simulink model "PID_Loop_2024a"  (R2024b)
settings: Solver=FixedStepAuto  StartTime=0.0  StopTime=tspan  FixedStep=dt  RelTol=1e-3
model workspace (MAT data in the model file):
  Drag_Constants = 1
  mass = [5.51 5.51 5.51 1 1 1]
  mass_6a = [5 5 5 1 1 1]
values from neighbouring files (symbols this model uses):
  acc_bias_instability = 19e-6*9.81    (= 0.00018639)    [init.m]
  acc_noise = 60e-6*9.81    (= 0.0005886)    [init.m]
  acc_vel_rw = 0.02/sqrt(3600)    [init.m]
  do_bouyancy_flag = 1    [PID_testing_data_producer.m]    (also in init.m = 0)
  do_gravity_flag = 1    [PID_testing_data_producer.m]    (also in init.m = 0)
  do_imu_noise_flag = 0    [PID_testing_data_producer.m]    (also in init.m)
  dt = 0.001    [PID_testing_data_producer.m]    (also in init.m)
  Dt = 0.01    [init.m]
  g = 9.8067    [constants.m]    (also in constants.mat = 9.80665)
  gyro_bias_instability = 1.5/3600/360    (= 1.15740740741e-06)    [init.m]
  gyro_noise = 5e-3*2*pi/360    (= 8.72664625997e-05)    [init.m]
  gyro_rw = 0.16*2*pi/360/sqrt(3600)    [init.m]
  H = [1 0 0 ... (first row only)    [init.m]
  inverse_wrench = pinv(wrench)    [calculate_wrench.m]    (also in constants.m = geometry_properties.inverse_wrench; geometry_properties.mat = [0.09 0.09 -0.09 -0.09 0.353553390593 0.353553390593 0.35355)
  mag_noise = 0.1    [init.m]
  max_pitch_torque = norm(wrench*(F_max*[1 1 -1 -1 0 0 0 0]'))    [calculate_wrench.m]
  max_roll_torque = norm(wrench*(F_max*[1 -1 1 -1 0 0 0 0]'))    [calculate_wrench.m]
  max_yaw_torque = norm(wrench*(F_max*[0 0 0 0 -1 1 -1 1]'))    [calculate_wrench.m]
  pitch_force = [0         0         0         0    1.0000         0]    [constants.m]
  plot_dt = 0.01    [init.m]
  Q = diag([0.0001, 0.0001, 0.1])    [init.m]
  R = [.1 0 ... (first row only)    [init.m]
  roll_force = [0         0         0    0.5000         0         0]    [constants.m]
  states_desired = [x_des;E_des]    [init.m]
  volume = 0.0074    [constants.m]    (also in constants.mat = 0.0073741788)
  volume_center = [0, 0, 0.1]    [constants.m]    (also in constants.mat = [0 0 0.1])
  water_density = 997    [constants.m]    (also in constants.mat = 1000)
  waypoints = input_state_errors(:,i)    [PID_testing_data_producer.m]    (also in init.m = [0, 0, 0])
  wrench = eval(w)    [calculate_wrench.m]    (also in constants.m = geometry_properties.wrench; constants.mat = [0 0 0 0 -0.7071 -0.7071 -0.7071 -0.7071 0 0 0 0 ... (48 ele; geometry_properties.mat = [0 0 -1 0.22 0.25 0 0 0 -1 -0.22 0.25 0 ... (48 elements, 6x; wrench.m)
  x_force = [0.4100         0         0         0         0         0]    [constants.m]    (also in init2.m = [0.410000000000000	0	0	0	0	0])
  y_force = [0    0.5000         0         0         0         0]    [constants.m]    (also in init2.m = [0	0.500000000000000	0	0	0	0])
  yaw_force = [0         0         0         0         0    0.5000]    [constants.m]
  z_force = [0         0    1.2500         0         0         0]    [constants.m]
undefined symbols (not defined in the file or in its folder): E0_est, fractalcoef, IMU, P, v0_e_est, x0_e_est
libraries: slpidlib x4, mspsensorlib x2, shared6dof x1, simulink x1, sharedTrackingLibrary x1, uavutilslib x1
(part 1 of 2)
settings Model: Creator=zenyn  LastModifiedBy=vinso
settings DataIOCC: LoggingToFile=on
settings OptimizationCC: EnhancedBackFolding=on  PassReuseOutputArgsAs=Individual arguments  ZeroExternalMemoryAtStartup=off  ZeroInternalMemoryAtStartup=off  MaxStackSize=64  OptimizeBlockOrder=speed  DifferentSizesBufferReuse=on  OptimizationCustomize=off  EfficientTunableParamExpr=on
settings DebuggingCC: ParameterTunabilityLossMsg=error
settings SFSimCC: MATLABDynamicMemAlloc=off
settings RTWCC: Description=Embedded Coder  SystemTargetFile=ert.tlc  HardwareBoard=Robot Operating System 2 (ROS 2)  TLCOptions="-aInlineSetEventsForThisBaseRateFcn=TLC_FALSE -aSuppressMultiTaskScheduler=TLC_FALSE  -aRateBasedStepFcn=0"  TemplateMakefile=ert_default_tmf  Toolchain=Colcon Tools  TargetLang=C++
settings CodeAppCC: ForceParamTrailComments=on  IgnoreCustomStorageClasses=off  OperatorAnnotations=on  SimulinkDataObjDesc=on  SFDataObjDesc=on  InsertBlockDesc=on
settings ERTTargetCC: CodeInterfacePackaging=C++ class  InlinedParameterPlacement=Hierarchical  RootIOFormat=Structure reference  DynamicArrayContainerType=coder::array

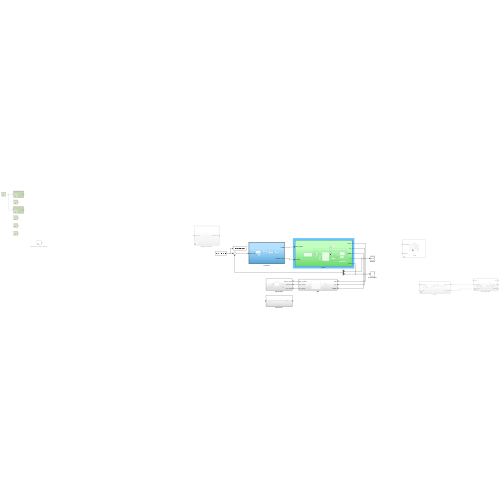
[thumbnail: Simulink's stored preview of the top-level diagram]
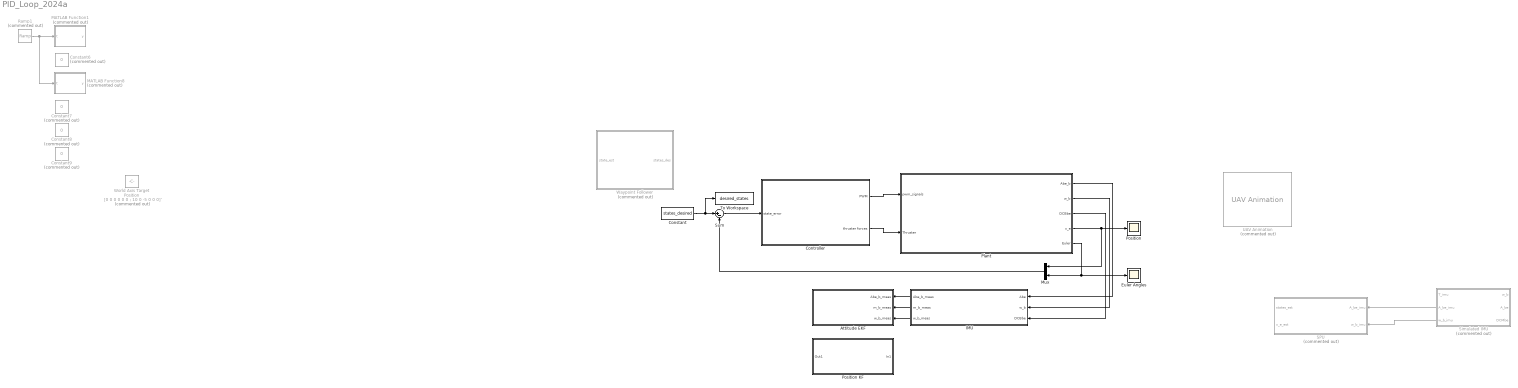
== system PID_Loop_2024a ==
  Attitude EKF : Subsystem
  Constant : Constant  Value=states_desired
  Constant{6..9} (4 alike) : Constant  Commented=on  Value=0
  Controller : Subsystem  TreatAsAtomicUnit=on
  Euler Angles : Scope
  IMU : Subsystem
  MATLAB Function1 : MATLAB Function  Commented=on  TreatAsAtomicUnit=on
  MATLAB Function8 : MATLAB Function  Commented=on  TreatAsAtomicUnit=on
  Mux : Mux  Inputs=2
  Plant : Subsystem
  Position : Scope
  Position KF : Subsystem
  Ramp1 : simulink/Sources/Ramp  Commented=on  slope=1  start=0  InitialOutput=0
  SPU : Subsystem  Commented=on
  Simulated IMU : Subsystem  Commented=on
  Sum : Sum  Inputs=|+-
  To Workspace : ToWorkspace  VariableName=desired_states  SaveFormat=Timeseries  SampleTime=Dt
  UAV Animation : uavutilslib/UAV Animation  Commented=on  NumUAV=1  DynamicUAVConfig=off  UAVType=FixedWing  UAVSize=1  UAVColor=[1 0 0]  UAVTrajectoryAlpha=1  InertialZDirection=Down  RotationFormat=Quaternion  DrawMarkers=off  SampleTime=Dt
  Waypoint Follower : Subsystem  Commented=on
  World Axis Target Position : Constant  Commented=on  Value=[0 0 0 0 0 0 ; 10 0 -5 0 0 0]'
  wires:
  Ramp1/1 -> MATLAB Function8/1(t), MATLAB Function1/1(t)
  Simulated IMU/2(A_be_imu) -> SPU/1(A_be_imu)
  Simulated IMU/3(w_b_imu) -> SPU/2(w_b_imu)
  Constant/1 -> Sum/1, To Workspace/1
  Plant/4(x_e) -> Position/1, Mux/1
  Sum/1 -> Controller/1(state_error)
  IMU/1(Abe_b_meas) -> Attitude EKF/1(Abe_b_meas)
  IMU/2(m_b_meas) -> Attitude EKF/2(m_b_meas)
  IMU/3(w_b_meas) -> Attitude EKF/3(w_b_meas)
  Plant/1(Abe_b) -> IMU/1(Abe)
  Plant/3(DCBbe) -> IMU/3(DCBbe)
  Plant/2(w_b) -> IMU/2(w_b)
  Controller/2(thruster forces) -> Plant/2(Thruster)
  Controller/1(PWM) -> Plant/1(pwm_signals)
  Plant/5(Euler) -> Mux/2, Euler Angles/1
  Mux/1 -> Sum/2

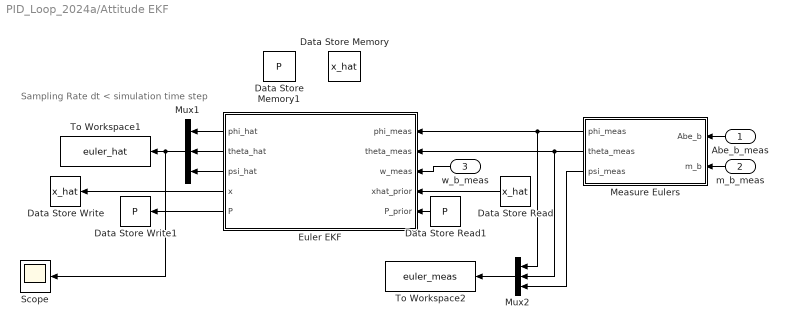
== system PID_Loop_2024a/Attitude EKF ==
  note: Sampling Rate dt < simulation time step
  Abe_b_meas : Inport
  m_b_meas : Inport  Port=2
  w_b_meas : Inport  Port=3
  Data Store Memory : DataStoreMemory  DataStoreName=x_hat  WriteAfterWriteMsg=warning  InitialValue=xhat0  ShowAdditionalParam=off
  Data Store Memory1 : DataStoreMemory  DataStoreName=P  WriteAfterWriteMsg=warning  InitialValue=P0  ShowAdditionalParam=off
  Data Store Read : DataStoreRead  DataStoreName=x_hat  IndexOptions=Index vector (dialog)  Indices=1  OutputSizes=1
  Data Store Read1 : DataStoreRead  DataStoreName=P  IndexOptions=Index vector (dialog)  Indices=1  OutputSizes=1
  Data Store Write : DataStoreWrite  DataStoreName=x_hat  IndexOptions=Index vector (dialog)  Indices=1  OutputSizes=1
  Data Store Write1 : DataStoreWrite  DataStoreName=P  IndexOptions=Index vector (dialog)  Indices=1  OutputSizes=1
  Euler EKF : MATLAB Function  TreatAsAtomicUnit=on
  Measure Eulers : MATLAB Function  TreatAsAtomicUnit=on
  Mux1 : Mux  Inputs=3
  Mux2 : Mux  Inputs=3
  Scope : Scope
  To Workspace1 : ToWorkspace  VariableName=euler_hat  SaveFormat=Timeseries  SampleTime=plot_dt
  To Workspace2 : ToWorkspace  VariableName=euler_meas  SaveFormat=Timeseries  SampleTime=plot_dt
  wires:
  Measure Eulers/1(phi_meas) -> Euler EKF/1(phi_meas), Mux2/1
  Euler EKF/4(x) -> Data Store Write/1
  Measure Eulers/2(theta_meas) -> Mux2/2, Euler EKF/2(theta_meas)
  Mux1/1 -> Scope/1, To Workspace1/1
  Data Store Read1/1 -> Euler EKF/5(P_prior)
  Euler EKF/1(phi_hat) -> Mux1/1
  Euler EKF/5(P) -> Data Store Write1/1
  Euler EKF/3(psi_hat) -> Mux1/3
  Euler EKF/2(theta_hat) -> Mux1/2
  Data Store Read/1 -> Euler EKF/4(xhat_prior)
  Abe_b_meas/1 -> Measure Eulers/1(Abe_b)
  Measure Eulers/3(psi_meas) -> Mux2/3
  Mux2/1 -> To Workspace2/1
  m_b_meas/1 -> Measure Eulers/2(m_b)
  w_b_meas/1 -> Euler EKF/3(w_meas)

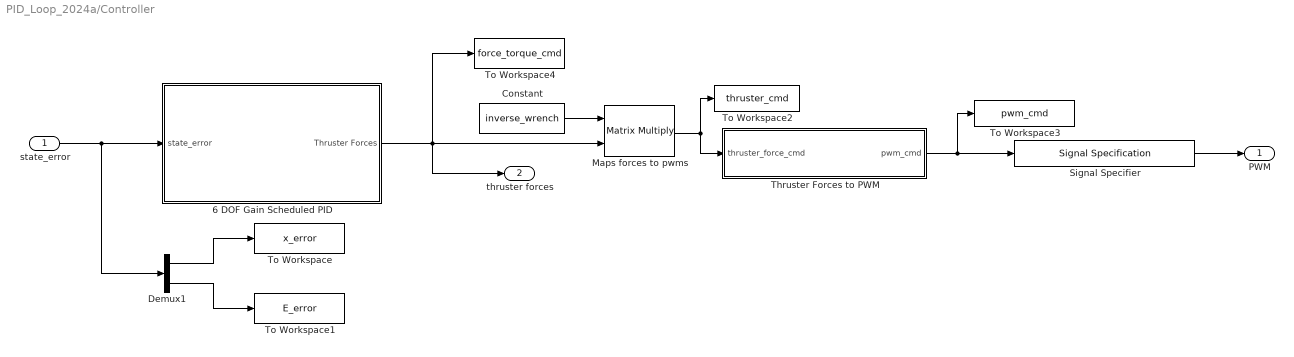
== system PID_Loop_2024a/Controller ==
  state_error : Inport
  6 DOF Gain Scheduled PID : Subsystem
  Constant : Constant  Value=inverse_wrench
  Demux1 : Demux  Outputs=2
  Maps forces to pwms : Product  Multiplication=Matrix(*)
  Signal Specifier : SignalSpecification  OutMin=[1200 ]  OutMax=[ 1800 ]  OutDataTypeStr=double  Unit=µs  Dimensions=[8 1]
  Thruster Forces to PWM : MATLAB Function  TreatAsAtomicUnit=on
  To Workspace : ToWorkspace  VariableName=x_error  SaveFormat=Timeseries  SampleTime=plot_dt
  To Workspace1 : ToWorkspace  VariableName=E_error  SaveFormat=Timeseries  SampleTime=plot_dt
  To Workspace2 : ToWorkspace  VariableName=thruster_cmd  SaveFormat=Timeseries  SampleTime=-1
  To Workspace3 : ToWorkspace  VariableName=pwm_cmd  SaveFormat=Timeseries  SampleTime=-1
  To Workspace4 : ToWorkspace  VariableName=force_torque_cmd  SaveFormat=Timeseries  SampleTime=plot_dt
  PWM : Outport
  thruster forces : Outport  Port=2
  wires:
  Thruster Forces to PWM/1(pwm_cmd) -> Signal Specifier/1, To Workspace3/1
  Signal Specifier/1 -> PWM/1
  Demux1/1 -> To Workspace/1
  Demux1/2 -> To Workspace1/1
  Maps forces to pwms/1 -> Thruster Forces to PWM/1(thruster_force_cmd), To Workspace2/1
  Constant/1 -> Maps forces to pwms/1
  state_error/1 -> 6 DOF Gain Scheduled PID/1(state_error), Demux1/1
  6 DOF Gain Scheduled PID/1(Thruster Forces) -> Maps forces to pwms/2, thruster forces/1, To Workspace4/1

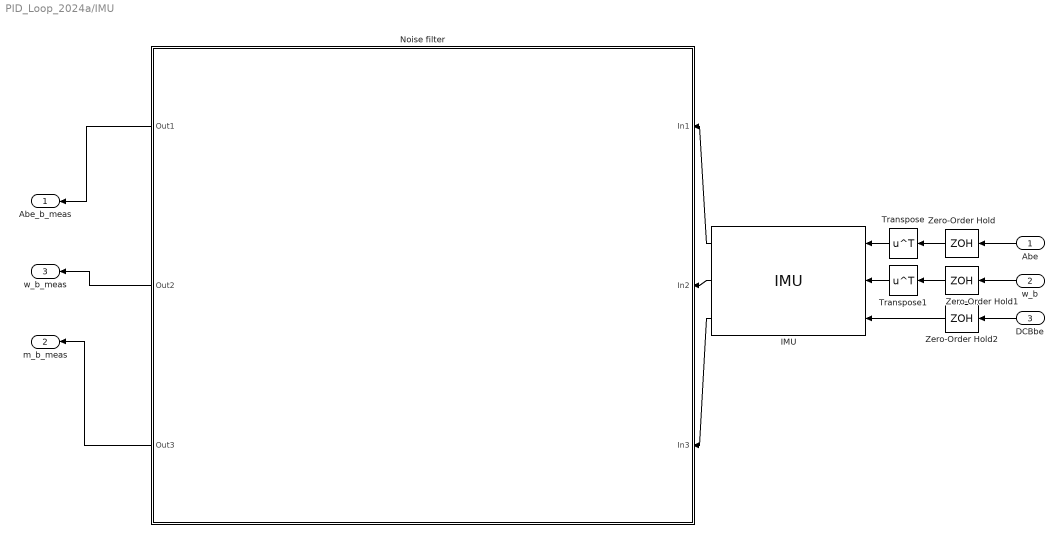
== system PID_Loop_2024a/IMU ==
  Abe : Inport
  w_b : Inport  Port=2
  DCBbe : Inport  Port=3
  IMU : mspsensorlib/IMU  DispRefFrame=NED  TemperaturePort=off  Temperature=25  MagneticFieldPort=off  MagneticFieldNED=[ 27.5550, -2.4169, -16.0849 ]  MagneticFieldENU=[ -2.4169, 27.5550, 16.0849 ]  SeedDouble=67  SimulateUsing=Interpreted execution  AccelParamsMeasurementRange=Inf  AccelParamsResolution=0  AccelParamsConstantBias=[ 0, 0, 0 ]  AccelParamsAxesMisalignment=[ 100, 0, 0; 0, 100, 0; 0, 0, 100 ]  AccelParamsNoiseDensity=acc_vel_rw*[ 1, 1, 1 ]  AccelParamsBiasInstability=acc_bias_instability*[ 1, 1, 1 ]  AccelParamsBiasInstabilityNumerator=fractalcoef().Numerator  AccelParamsBiasInstabilityDenominator=fractalcoef().Denominator  AccelParamsRandomWalk=acc_noise*[1, 1, 1]  AccelParamsNoiseType=double-sided  AccelParamsTemperatureBias=[ 0, 0, 0 ]  AccelParamsTemperatureScaleFactor=[ 0, 0, 0 ]  GyroParamsMeasurementRange=Inf  GyroParamsResolution=0  GyroParamsConstantBias=[ 0, 0, 0 ]  GyroParamsAxesMisalignment=[ 100, 0, 0; 0, 100, 0; 0, 0, 100 ]  GyroParamsAccelerationBias=[ 0, 0, 0 ]  GyroParamsNoiseDensity=gyro_rw*[ 1, 1, 1 ]  GyroParamsBiasInstability=gyro_bias_instability*[ 1, 1, 1 ]  GyroParamsBiasInstabilityNumerator=fractalcoef().Numerator  GyroParamsBiasInstabilityDenominator=fractalcoef().Denominator  GyroParamsRandomWalk=gyro_noise*[1, 1, 1]  GyroParamsNoiseType=double-sided  GyroParamsTemperatureBias=[ 0, 0, 0 ]  GyroParamsTemperatureScaleFactor=[ 0, 0, 0 ]  MagParamsMeasurementRange=Inf  MagParamsResolution=0  MagParamsConstantBias=[ 0, 0, 0 ]  MagParamsAxesMisalignment=[ 100, 0, 0; 0, 100, 0; 0, 0, 100 ]  MagParamsNoiseDensity=mag_noise*[1, 1, 1]  MagParamsBiasInstability=[ 0, 0, 0 ]  MagParamsBiasInstabilityNumerator=fractalcoef().Numerator  MagParamsBiasInstabilityDenominator=fractalcoef().Denominator  MagParamsRandomWalk=[ 0, 0, 0 ]  MagParamsNoiseType=double-sided  MagParamsTemperatureBias=[ 0, 0, 0 ]  MagParamsTemperatureScaleFactor=[ 0, 0, 0 ]
  Noise filter : Subsystem
  Transpose : Math  Operator=transpose
  Transpose1 : Math  Operator=transpose
  Zero-Order Hold : ZeroOrderHold  SampleTime=dt
  Zero-Order Hold1 : ZeroOrderHold  SampleTime=dt
  Zero-Order Hold2 : ZeroOrderHold  SampleTime=dt
  Abe_b_meas : Outport
  m_b_meas : Outport  Port=2
  w_b_meas : Outport  Port=3
  wires:
  Transpose/1 -> IMU/1
  Zero-Order Hold2/1 -> IMU/3
  Zero-Order Hold/1 -> Transpose/1
  Transpose1/1 -> IMU/2
  Zero-Order Hold1/1 -> Transpose1/1
  w_b/1 -> Zero-Order Hold1/1
  Abe/1 -> Zero-Order Hold/1
  DCBbe/1 -> Zero-Order Hold2/1
  IMU/1 -> Noise filter/1(In1)
  IMU/2 -> Noise filter/2(In2)
  IMU/3 -> Noise filter/3(In3)
  Noise filter/1(Out1) -> Abe_b_meas/1
  Noise filter/2(Out2) -> w_b_meas/1
  Noise filter/3(Out3) -> m_b_meas/1

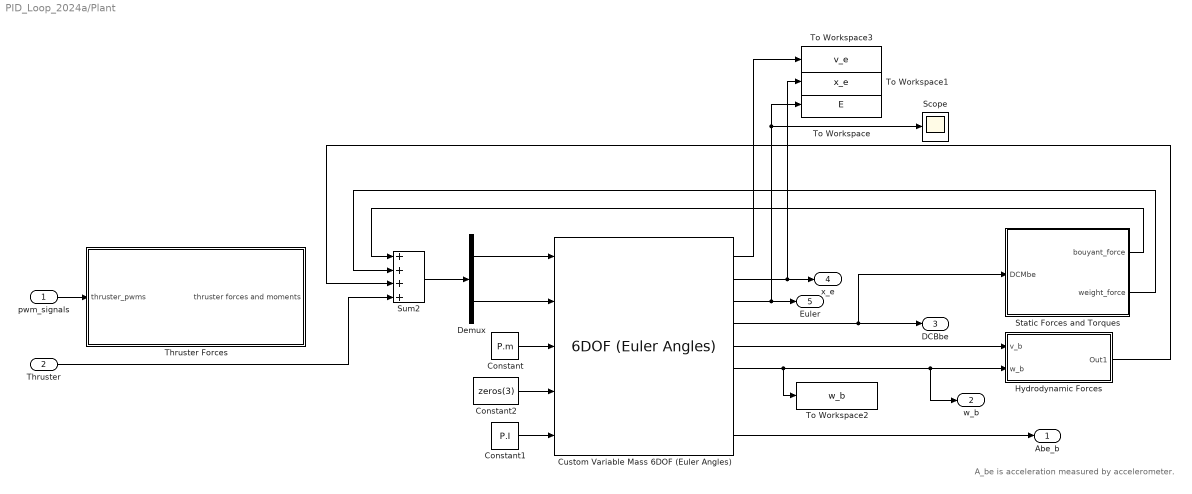
== system PID_Loop_2024a/Plant ==
  note: A_be is acceleration measured by accelerometer.
  pwm_signals : Inport  SampleTime=dt
  Thruster : Inport  Port=2
  Constant : Constant  Value=P.m
  Constant1 : Constant  Value=P.I
  Constant2 : Constant  Value=zeros(3)
  Custom Variable Mass 6DOF (Euler Angles) : shared6dof/6DOF (Euler Angles)  units=Metric (MKS)  mtype=Custom Variable  rep=Euler Angles  xme_0=x0_e  Vm_0=v0_e  eul_0=E0  pm_0=w0  mass_0=1.0  mass_e=0.5  mass_f=2.0  inertia=eye(3)  inertia_e=eye(3)  inertia_f=2*eye(3)  k_quat=1.0  vre_flag=off  abi_flag=on  aMode=0  xme_statename=''  Vm_statename=''  eul_statename=''  quat_statename=''  pm_statename=''  mass_statename=''
      settings: LibrarySourceBlock=aerolib6dof2/Custom Variable Mass 6DOF (Euler Angles)
  Demux : Demux  Outputs=2
  Hydrodynamic Forces : Subsystem
  Scope : Scope
  Static Forces and Torques : Subsystem
  Sum2 : Sum  Inputs=++++
  Thruster Forces : Subsystem
  To Workspace : ToWorkspace  VariableName=E  SaveFormat=Timeseries  SampleTime=plot_dt
  To Workspace1 : ToWorkspace  VariableName=x_e  SaveFormat=Timeseries  SampleTime=plot_dt
  To Workspace2 : ToWorkspace  VariableName=w_b  SaveFormat=Timeseries  SampleTime=plot_dt
  To Workspace3 : ToWorkspace  VariableName=v_e  SaveFormat=Timeseries  SampleTime=plot_dt
  Abe_b : Outport  SampleTime=Dt
  w_b : Outport  Port=2  SampleTime=Dt
  DCBbe : Outport  Port=3  SampleTime=Dt
  x_e : Outport  Port=4
  Euler : Outport  Port=5
  wires:
  Custom Variable Mass 6DOF (Euler Angles)/9 -> Abe_b/1
  Constant/1 -> Custom Variable Mass 6DOF (Euler Angles)/3
  Constant1/1 -> Custom Variable Mass 6DOF (Euler Angles)/5
  Constant2/1 -> Custom Variable Mass 6DOF (Euler Angles)/4
  Custom Variable Mass 6DOF (Euler Angles)/5 -> Hydrodynamic Forces/1(v_b)
  Custom Variable Mass 6DOF (Euler Angles)/4 -> Static Forces and Torques/1(DCMbe), DCBbe/1
  pwm_signals/1 -> Thruster Forces/1(thruster_pwms)
  Hydrodynamic Forces/1(Out1) -> Sum2/3
  Static Forces and Torques/2(weight_force) -> Sum2/2
  Static Forces and Torques/1(bouyant_force) -> Sum2/1
  Custom Variable Mass 6DOF (Euler Angles)/6 -> To Workspace2/1, w_b/1, Hydrodynamic Forces/2(w_b)
  Demux/2 -> Custom Variable Mass 6DOF (Euler Angles)/2
  Demux/1 -> Custom Variable Mass 6DOF (Euler Angles)/1
  Custom Variable Mass 6DOF (Euler Angles)/3 -> Euler/1, Scope/1, To Workspace/1
  Custom Variable Mass 6DOF (Euler Angles)/2 -> To Workspace1/1, x_e/1
  Custom Variable Mass 6DOF (Euler Angles)/1 -> To Workspace3/1
  Sum2/1 -> Demux/1
  Thruster/1 -> Sum2/4

== system PID_Loop_2024a/Position KF ==
  In1 : Inport
  Out1 : Outport
  wires:
  In1/1 -> Out1/1

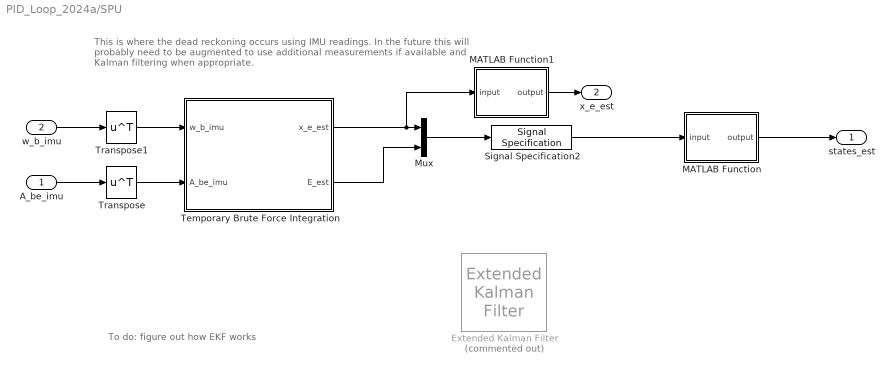
== system PID_Loop_2024a/SPU ==
  note: To do: figure out how EKF works
  note: This is where the dead reckoning occurs using IMU readings. In the future this will
      | probably need to be augmented to use additional measurements if available and
      | Kalman filtering when appropriate.
  A_be_imu : Inport
  w_b_imu : Inport  Port=2
  Extended Kalman Filter : sharedTrackingLibrary/Extended Kalman Filter  Commented=on  StateTransitionFcn=myStateTransitionFcn  HasStateTransitionJacobianFcn=off  HasAdditiveProcessNoise=Additive  ProcessNoise=1  HasTimeVaryingProcessNoise=off  HasStateTransitionFcnExtraArgument=0  InitialState=0  InitialStateCovariance=1  MeasurementFcn1=myMeasurementFcn  HasMeasurementJacobianFcn1=off  HasMeasurementEnablePort1=off  HasAdditiveMeasurementNoise1=Additive  MeasurementNoise1=1  HasTimeVaryingMeasurementNoise1=off  HasMeasurementFcnExtraArgument1=0  HasMeasurementWrapping1=off  MeasurementFcn2=myMeasurementFcn  HasMeasurementJacobianFcn2=off  HasMeasurementEnablePort2=off  HasAdditiveMeasurementNoise2=Additive  MeasurementNoise2=1  HasTimeVaryingMeasurementNoise2=off  HasMeasurementFcnExtraArgument2=0  HasMeasurementWrapping2=off  MeasurementFcn3=myMeasurementFcn  HasMeasurementJacobianFcn3=off  HasMeasurementEnablePort3=off  HasAdditiveMeasurementNoise3=Additive  MeasurementNoise3=1  HasTimeVaryingMeasurementNoise3=off  HasMeasurementFcnExtraArgument3=0  HasMeasurementWrapping3=off  MeasurementFcn4=myMeasurementFcn  HasMeasurementJacobianFcn4=off  HasMeasurementEnablePort4=off  HasAdditiveMeasurementNoise4=Additive  MeasurementNoise4=1  HasTimeVaryingMeasurementNoise4=off  HasMeasurementFcnExtraArgument4=0  HasMeasurementWrapping4=off  MeasurementFcn5=myMeasurementFcn  HasMeasurementJacobianFcn5=off  HasMeasurementEnablePort5=off  HasAdditiveMeasurementNoise5=Additive  MeasurementNoise5=1  HasTimeVaryingMeasurementNoise5=off  HasMeasurementFcnExtraArgument5=0  HasMeasurementWrapping5=off  EnableMultirate=off  StateTransitionFcnSampleTime=1  MeasurementFcn1SampleTime=1  MeasurementFcn2SampleTime=1  MeasurementFcn3SampleTime=1  MeasurementFcn4SampleTime=1  MeasurementFcn5SampleTime=1  UseCurrentEstimator=on  OutputStateCovariance=off  DataType=double  SampleTime=1  NumberOfMeasurements=1
  MATLAB Function : MATLAB Function  TreatAsAtomicUnit=on
  MATLAB Function1 : MATLAB Function  TreatAsAtomicUnit=on
  Mux : Mux  Inputs=2
  Signal Specification2 : SignalSpecification  Dimensions=[6 1]
  Temporary Brute Force Integration : Subsystem
  Transpose : Math  Operator=transpose
  Transpose1 : Math  Operator=transpose
  states_est : Outport
  x_e_est : Outport  Port=2
  wires:
  w_b_imu/1 -> Transpose1/1
  A_be_imu/1 -> Transpose/1
  Temporary Brute Force Integration/2(E_est) -> Mux/2
  Temporary Brute Force Integration/1(x_e_est) -> MATLAB Function1/1(input), Mux/1
  Mux/1 -> Signal Specification2/1
  Signal Specification2/1 -> MATLAB Function/1(input)
  Transpose1/1 -> Temporary Brute Force Integration/1(w_b_imu)
  Transpose/1 -> Temporary Brute Force Integration/2(A_be_imu)
  MATLAB Function/1(output) -> states_est/1
  MATLAB Function1/1(output) -> x_e_est/1

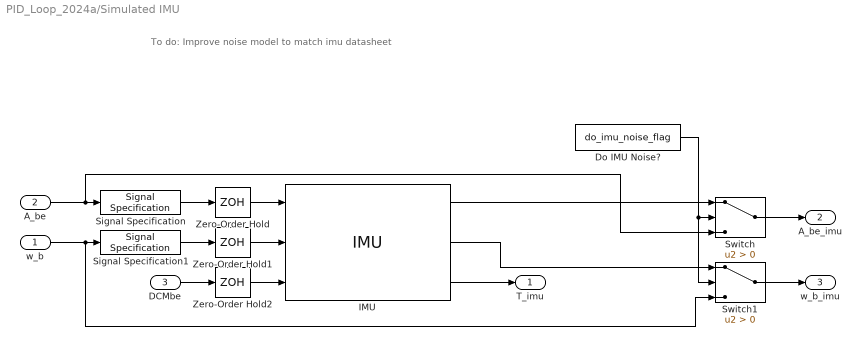
== system PID_Loop_2024a/Simulated IMU ==
  note: To do: Improve noise model to match imu datasheet
  w_b : Inport  SampleTime=Dt
  A_be : Inport  Port=2  SampleTime=Dt
  DCMbe : Inport  Port=3
  Do IMU Noise? : Constant  Value=do_imu_noise_flag
  IMU : mspsensorlib/IMU  DispRefFrame=NED  TemperaturePort=off  Temperature=25  MagneticFieldPort=off  MagneticFieldNED=[ 27.5550, -2.4169, -16.0849 ]  MagneticFieldENU=[ -2.4169, 27.5550, 16.0849 ]  SeedDouble=67  SimulateUsing=Interpreted execution  AccelParamsMeasurementRange=IMU.accelMaxRating  AccelParamsResolution=IMU.accelResolution  AccelParamsConstantBias=[ 0, 0, 0 ]  AccelParamsAxesMisalignment=[ 100, 0, 0; 0, 100, 0; 0, 0, 100 ]  AccelParamsNoiseDensity=[ IMU.accelVelRNDWalk, 0, 0 ]  AccelParamsBiasInstability=[ 0, 0, 0 ]  AccelParamsBiasInstabilityNumerator=fractalcoef().Numerator  AccelParamsBiasInstabilityDenominator=fractalcoef().Denominator  AccelParamsRandomWalk=[ 0, 0, 0 ]  AccelParamsNoiseType=double-sided  AccelParamsTemperatureBias=[ 0, 0, 0 ]  AccelParamsTemperatureScaleFactor=[ 0, 0, 0 ]  GyroParamsMeasurementRange=Inf  GyroParamsResolution=IMU.gyroResolution  GyroParamsConstantBias=[ 0, 0, 0 ]  GyroParamsAxesMisalignment=[ 100, 0, 0; 0, 100, 0; 0, 0, 100 ]  GyroParamsAccelerationBias=[ 0, 0, 0 ]  GyroParamsNoiseDensity=[ IMU.gyroAngleRNDWalk, 0, 0 ]  GyroParamsBiasInstability=[ 0, 0, 0 ]  GyroParamsBiasInstabilityNumerator=fractalcoef().Numerator  GyroParamsBiasInstabilityDenominator=fractalcoef().Denominator  GyroParamsRandomWalk=[ 0, 0, 0 ]  GyroParamsNoiseType=double-sided  GyroParamsTemperatureBias=[ 0, 0, 0 ]  GyroParamsTemperatureScaleFactor=[ 0, 0, 0 ]  MagParamsMeasurementRange=Inf  MagParamsResolution=IMU.magsResolution  MagParamsConstantBias=[ 0, 0, 0 ]  MagParamsAxesMisalignment=[ 100, 0, 0; 0, 100, 0; 0, 0, 100 ]  MagParamsNoiseDensity=[ 0, 0, 0 ]  MagParamsBiasInstability=[ 0, 0, 0 ]  MagParamsBiasInstabilityNumerator=fractalcoef().Numerator  MagParamsBiasInstabilityDenominator=fractalcoef().Denominator  MagParamsRandomWalk=[ 0, 0, 0 ]  MagParamsNoiseType=double-sided  MagParamsTemperatureBias=[ 0, 0, 0 ]  MagParamsTemperatureScaleFactor=[ 0, 0, 0 ]
  Signal Specification : SignalSpecification  Dimensions=[1 3]
  Signal Specification1 : SignalSpecification  Dimensions=[1 3]
  Switch : Switch  Criteria=u2 > Threshold  SaturateOnIntegerOverflow=off  InputSameDT=off
  Switch1 : Switch  Criteria=u2 > Threshold  SaturateOnIntegerOverflow=off  InputSameDT=off
  Zero-Order Hold : ZeroOrderHold  SampleTime=Dt
  Zero-Order Hold1 : ZeroOrderHold  SampleTime=Dt
  Zero-Order Hold2 : ZeroOrderHold  SampleTime=Dt
  T_imu : Outport
  A_be_imu : Outport  Port=2
  w_b_imu : Outport  Port=3
  wires:
  w_b/1 -> Switch1/3, Signal Specification1/1
  A_be/1 -> Switch/3, Signal Specification/1
  Signal Specification/1 -> Zero-Order Hold/1
  Signal Specification1/1 -> Zero-Order Hold1/1
  IMU/1 -> Switch/1
  IMU/2 -> Switch1/1
  IMU/3 -> T_imu/1
  DCMbe/1 -> Zero-Order Hold2/1
  Zero-Order Hold/1 -> IMU/1
  Zero-Order Hold1/1 -> IMU/2
  Zero-Order Hold2/1 -> IMU/3
  Do IMU Noise?/1 -> Switch1/2, Switch/2
  Switch/1 -> A_be_imu/1
  Switch1/1 -> w_b_imu/1

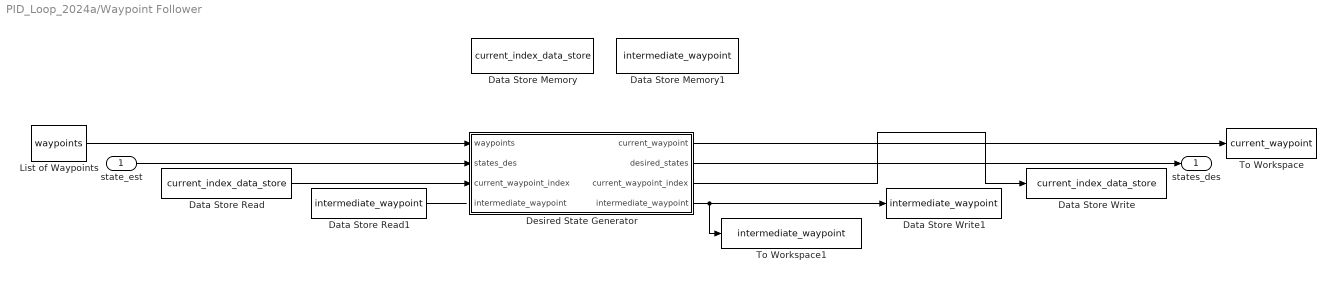
== system PID_Loop_2024a/Waypoint Follower ==
  state_est : Inport  SampleTime=Dt
  Data Store Memory : DataStoreMemory  DataStoreName=current_index_data_store  WriteAfterWriteMsg=warning  InitialValue=1  ShowAdditionalParam=off
  Data Store Memory1 : DataStoreMemory  DataStoreName=intermediate_waypoint  WriteAfterWriteMsg=warning  InitialValue=[9999,9999,9999]  ShowAdditionalParam=off
  Data Store Read : DataStoreRead  DataStoreName=current_index_data_store  IndexOptions=Index vector (dialog)  Indices=1  OutputSizes=1
  Data Store Read1 : DataStoreRead  DataStoreName=intermediate_waypoint  IndexOptions=Index vector (dialog)  Indices=1  OutputSizes=1
  Data Store Write : DataStoreWrite  DataStoreName=current_index_data_store  IndexOptions=Index vector (dialog)  Indices=1  OutputSizes=1
  Data Store Write1 : DataStoreWrite  DataStoreName=intermediate_waypoint  IndexOptions=Index vector (dialog)  Indices=1  OutputSizes=1
  Desired State Generator : MATLAB Function  TreatAsAtomicUnit=on
  List of Waypoints : Constant  Value=waypoints
  To Workspace : ToWorkspace  VariableName=current_waypoint  SaveFormat=Timeseries  SampleTime=-1
  To Workspace1 : ToWorkspace  VariableName=intermediate_waypoint  SaveFormat=Timeseries  SampleTime=-1
  states_des : Outport  SampleTime=Dt
  wires:
  state_est/1 -> Desired State Generator/2(states_des)
  Desired State Generator/2(desired_states) -> states_des/1
  Desired State Generator/3(current_waypoint_index) -> Data Store Write/1
  List of Waypoints/1 -> Desired State Generator/1(waypoints)
  Desired State Generator/1(current_waypoint) -> To Workspace/1
  Data Store Read/1 -> Desired State Generator/3("current_waypoint_index ")
  Data Store Read1/1 -> ?
  Desired State Generator/4(intermediate_waypoint) -> Data Store Write1/1, To Workspace1/1
  ? -> Desired State Generator/4("intermediate_waypoint ")

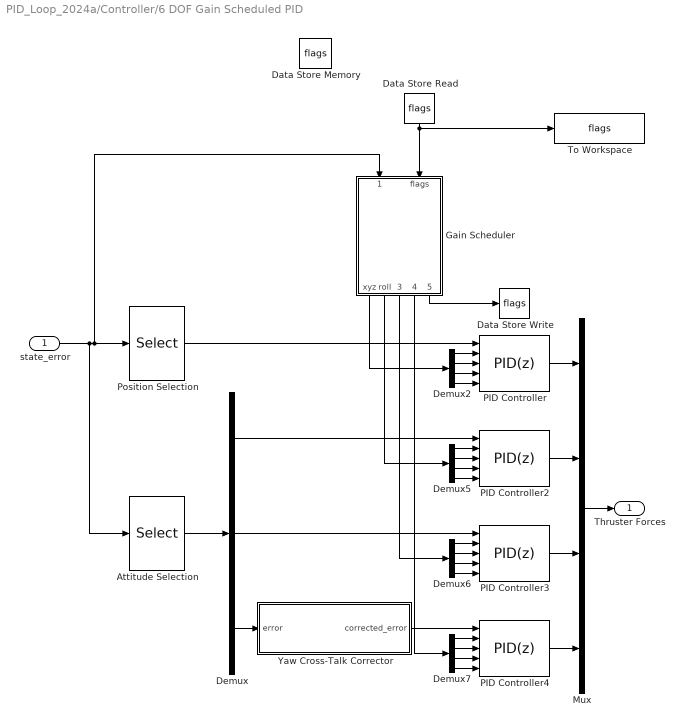
== system PID_Loop_2024a/Controller/6 DOF Gain Scheduled PID ==
  state_error : Inport  SampleTime=Dt
  Attitude Selection : Selector  InputPortWidth=6  IndexOptions=Index vector (dialog)  Indices=[4:6]  OutputSizes=1
  Data Store Memory : DataStoreMemory  DataStoreName=flags  WriteAfterWriteMsg=warning  InitialValue=[1 1 0]  ShowAdditionalParam=off
  Data Store Read : DataStoreRead  DataStoreName=flags  IndexOptions=Index vector (dialog)  Indices=1  OutputSizes=1
  Data Store Write : DataStoreWrite  DataStoreName=flags  IndexOptions=Index vector (dialog)  Indices=1  OutputSizes=1
  Demux : Demux  Outputs=3
  Demux{2,5..7} (4 alike) : Demux
  Gain Scheduler : MATLAB Function  TreatAsAtomicUnit=on
  Mux : Mux
  PID Controller : slpidlib/PID Controller  Controller=PID  Form=Parallel  TimeDomain=Discrete-time  UseExternalTs=off  SampleTime=-1  IntegratorMethod=Forward Euler  FilterMethod=Forward Euler  ControllerParametersSource=external  P=18.567926327114  I=2.74882046275699  UseKiTs=off  D=30.7980856287723  UseExternalDerivativeSource=off  N=17.2469682941307  UseFilter=on  TunerSelectOption=Transfer Function Based (PID Tuner App)  InitialConditionSource=internal  InitialConditionForIntegrator=0  InitialConditionForFilter=0  DifferentiatorICPrevScaledInput=0  ExternalReset=none  TrackingMode=off  Kt=1  LimitOutput=on  SatLimitsSource=internal  UpperSaturationLimit=80  LowerSaturationLimit=-80  LinearizeAsGain=on  AntiWindupMode=none  Kb=1  LimitIntegrator=off  UpperIntegratorSaturationLimit=inf  LowerIntegratorSaturationLimit=-inf  POutMin=[]  POutMax=[]  IOutMin=[]  IOutMax=[]  DOutMin=[]  DOutMax=[]  NOutMin=[]  NOutMax=[]  SumOutMin=[]  SumOutMax=[]  SaturationOutMin=[]  SaturationOutMax=[]  PParamMin=[]  PParamMax=[]  IParamMin=[]  IParamMax=[]  DParamMin=[]  DParamMax=[]  NParamMin=[]  NParamMax=[]  KbParamMin=[]  KbParamMax=[]  KtParamMin=[]  KtParamMax=[]  KbOutMin=[]  KbOutMax=[]  KtOutMin=[]  KtOutMax=[]  IntegratorOutMin=[]  IntegratorOutMax=[]  FilterOutMin=[]  FilterOutMax=[]  SumI1OutMin=[]  SumI1OutMax=[]  SumI2OutMin=[]  SumI2OutMax=[]  SumI3OutMin=[]  SumI3OutMax=[]  SumI4OutMin=[]  SumI4OutMax=[]  SumDOutMin=[]  SumDOutMax=[]  DifferentiatorOutMin=[]  DifferentiatorOutMax=[]  FilterDiffOutCoefMin=[]  FilterDiffOutCoefMax=[]  ReciprocalOutMin=[]  ReciprocalOutMax=[]  SumDenOutMin=[]  SumDenOutMax=[]  SumNumOutMin=[]  SumNumOutMax=[]  DivideOutMin=[]  DivideOutMax=[]  UdiffTsProdOutMin=[]  UdiffTsProdOutMax=[]  NTsProdOutMin=[]  NTsProdOutMax=[]  UintegralTsProdOutMin=[]  UintegralTsProdOutMax=[]  UngainTsProdOutMin=[]  UngainTsProdOutMax=[]  ClampingZeroOutDataTypeStr=Inherit: Inherit via back propagation  ClampingZeroOutMin=[]  ClampingZeroOutMax=[]  FilterDenConstantOutDataTypeStr=Inherit: Inherit via back propagation  FilterDenConstantOutMin=[]  FilterDenConstantOutMax=[]  PCopyOutDataTypeStr=Inherit: Inherit via back propagation  PCopyOutMin=[]  PCopyOutMax=[]  NCopyOutDataTypeStr=Inherit: Inherit via back propagation  NCopyOutMin=[]  NCopyOutMax=[]  IntegratorContinuousStateAttributes=''  IntegratorStateMustResolveToSignalObject=off  IntegratorRTWStateStorageClass=Auto  FilterContinuousStateAttributes=''  FilterStateMustResolveToSignalObject=off  FilterRTWStateStorageClass=Auto  ParallelPVariant=ExternalParameters  IdealPVariant=Disabled  IVariant=ExternalParameters  DVariant=ExternalParameters  IntegratorVariant=Discrete  SatVariant=Enabled  AWVariant=Passthrough  PCopyVariant=Disabled  TRVariant=Disabled  FdbkBlocksVariant=Forward  IdealPFdbkVariant=Disabled  SatFdbkVariant=Disabled  DerivativeFilterVariant=ForwardEulerFilter  NVariant=ExternalParameters  NCopyVariant=Disabled  FilterICVariant=InternalICsFilter  IntegratorICVariant=InternalICs  ExternalResetVariant=Disabled  TRSumVariant=Passthrough  SumFdbkVariant=Disabled  SumVariant=Sum_PID  TsampFilterVariant=InternalTs  TsampNgainVariant=Passthrough  TsampIntegralVariant=Disabled_SignalSpec  ExternalSaturationOutDataTypeStr=Inherit: Same as second input  DerivativeSourceVariant=ErrorSignal  PreIntVariant=InternalPreInt
  PID Controller2 : slpidlib/PID Controller  Controller=PID  Form=Parallel  TimeDomain=Discrete-time  UseExternalTs=off  SampleTime=-1  IntegratorMethod=Forward Euler  FilterMethod=Forward Euler  ControllerParametersSource=external  P=18.567926327114  I=2.74882046275699  UseKiTs=off  D=30.7980856287723  UseExternalDerivativeSource=off  N=17.2469682941307  UseFilter=on  TunerSelectOption=Transfer Function Based (PID Tuner App)  InitialConditionSource=internal  InitialConditionForIntegrator=0  InitialConditionForFilter=0  DifferentiatorICPrevScaledInput=0  ExternalReset=none  TrackingMode=off  Kt=1  LimitOutput=on  SatLimitsSource=internal  UpperSaturationLimit=max_roll_torque  LowerSaturationLimit=-max_roll_torque  LinearizeAsGain=on  AntiWindupMode=none  Kb=1  LimitIntegrator=off  UpperIntegratorSaturationLimit=inf  LowerIntegratorSaturationLimit=-inf  POutMin=[]  POutMax=[]  IOutMin=[]  IOutMax=[]  DOutMin=[]  DOutMax=[]  NOutMin=[]  NOutMax=[]  SumOutMin=[]  SumOutMax=[]  SaturationOutMin=[]  SaturationOutMax=[]  PParamMin=[]  PParamMax=[]  IParamMin=[]  IParamMax=[]  DParamMin=[]  DParamMax=[]  NParamMin=[]  NParamMax=[]  KbParamMin=[]  KbParamMax=[]  KtParamMin=[]  KtParamMax=[]  KbOutMin=[]  KbOutMax=[]  KtOutMin=[]  KtOutMax=[]  IntegratorOutMin=[]  IntegratorOutMax=[]  FilterOutMin=[]  FilterOutMax=[]  SumI1OutMin=[]  SumI1OutMax=[]  SumI2OutMin=[]  SumI2OutMax=[]  SumI3OutMin=[]  SumI3OutMax=[]  SumI4OutMin=[]  SumI4OutMax=[]  SumDOutMin=[]  SumDOutMax=[]  DifferentiatorOutMin=[]  DifferentiatorOutMax=[]  FilterDiffOutCoefMin=[]  FilterDiffOutCoefMax=[]  ReciprocalOutMin=[]  ReciprocalOutMax=[]  SumDenOutMin=[]  SumDenOutMax=[]  SumNumOutMin=[]  SumNumOutMax=[]  DivideOutMin=[]  DivideOutMax=[]  UdiffTsProdOutMin=[]  UdiffTsProdOutMax=[]  NTsProdOutMin=[]  NTsProdOutMax=[]  UintegralTsProdOutMin=[]  UintegralTsProdOutMax=[]  UngainTsProdOutMin=[]  UngainTsProdOutMax=[]  ClampingZeroOutDataTypeStr=Inherit: Inherit via back propagation  ClampingZeroOutMin=[]  ClampingZeroOutMax=[]  FilterDenConstantOutDataTypeStr=Inherit: Inherit via back propagation  FilterDenConstantOutMin=[]  FilterDenConstantOutMax=[]  PCopyOutDataTypeStr=Inherit: Inherit via back propagation  PCopyOutMin=[]  PCopyOutMax=[]  NCopyOutDataTypeStr=Inherit: Inherit via back propagation  NCopyOutMin=[]  NCopyOutMax=[]  IntegratorContinuousStateAttributes=''  IntegratorStateMustResolveToSignalObject=off  IntegratorRTWStateStorageClass=Auto  FilterContinuousStateAttributes=''  FilterStateMustResolveToSignalObject=off  FilterRTWStateStorageClass=Auto  ParallelPVariant=ExternalParameters  IdealPVariant=Disabled  IVariant=ExternalParameters  DVariant=ExternalParameters  IntegratorVariant=Discrete  SatVariant=Enabled  AWVariant=Passthrough  PCopyVariant=Disabled  TRVariant=Disabled  FdbkBlocksVariant=Forward  IdealPFdbkVariant=Disabled  SatFdbkVariant=Disabled  DerivativeFilterVariant=ForwardEulerFilter  NVariant=ExternalParameters  NCopyVariant=Disabled  FilterICVariant=InternalICsFilter  IntegratorICVariant=InternalICs  ExternalResetVariant=Disabled  TRSumVariant=Passthrough  SumFdbkVariant=Disabled  SumVariant=Sum_PID  TsampFilterVariant=InternalTs  TsampNgainVariant=Passthrough  TsampIntegralVariant=Disabled_SignalSpec  ExternalSaturationOutDataTypeStr=Inherit: Same as second input  DerivativeSourceVariant=ErrorSignal  PreIntVariant=InternalPreInt
  PID Controller3 : slpidlib/PID Controller  Controller=PID  Form=Parallel  TimeDomain=Discrete-time  UseExternalTs=off  SampleTime=-1  IntegratorMethod=Forward Euler  FilterMethod=Forward Euler  ControllerParametersSource=external  P=18.567926327114  I=2.74882046275699  UseKiTs=off  D=30.7980856287723  UseExternalDerivativeSource=off  N=17.2469682941307  UseFilter=on  TunerSelectOption=Transfer Function Based (PID Tuner App)  InitialConditionSource=internal  InitialConditionForIntegrator=0  InitialConditionForFilter=0  DifferentiatorICPrevScaledInput=0  ExternalReset=none  TrackingMode=off  Kt=1  LimitOutput=on  SatLimitsSource=internal  UpperSaturationLimit=max_pitch_torque  LowerSaturationLimit=-max_pitch_torque  LinearizeAsGain=on  AntiWindupMode=none  Kb=1  LimitIntegrator=off  UpperIntegratorSaturationLimit=inf  LowerIntegratorSaturationLimit=-inf  POutMin=[]  POutMax=[]  IOutMin=[]  IOutMax=[]  DOutMin=[]  DOutMax=[]  NOutMin=[]  NOutMax=[]  SumOutMin=[]  SumOutMax=[]  SaturationOutMin=[]  SaturationOutMax=[]  PParamMin=[]  PParamMax=[]  IParamMin=[]  IParamMax=[]  DParamMin=[]  DParamMax=[]  NParamMin=[]  NParamMax=[]  KbParamMin=[]  KbParamMax=[]  KtParamMin=[]  KtParamMax=[]  KbOutMin=[]  KbOutMax=[]  KtOutMin=[]  KtOutMax=[]  IntegratorOutMin=[]  IntegratorOutMax=[]  FilterOutMin=[]  FilterOutMax=[]  SumI1OutMin=[]  SumI1OutMax=[]  SumI2OutMin=[]  SumI2OutMax=[]  SumI3OutMin=[]  SumI3OutMax=[]  SumI4OutMin=[]  SumI4OutMax=[]  SumDOutMin=[]  SumDOutMax=[]  DifferentiatorOutMin=[]  DifferentiatorOutMax=[]  FilterDiffOutCoefMin=[]  FilterDiffOutCoefMax=[]  ReciprocalOutMin=[]  ReciprocalOutMax=[]  SumDenOutMin=[]  SumDenOutMax=[]  SumNumOutMin=[]  SumNumOutMax=[]  DivideOutMin=[]  DivideOutMax=[]  UdiffTsProdOutMin=[]  UdiffTsProdOutMax=[]  NTsProdOutMin=[]  NTsProdOutMax=[]  UintegralTsProdOutMin=[]  UintegralTsProdOutMax=[]  UngainTsProdOutMin=[]  UngainTsProdOutMax=[]  ClampingZeroOutDataTypeStr=Inherit: Inherit via back propagation  ClampingZeroOutMin=[]  ClampingZeroOutMax=[]  FilterDenConstantOutDataTypeStr=Inherit: Inherit via back propagation  FilterDenConstantOutMin=[]  FilterDenConstantOutMax=[]  PCopyOutDataTypeStr=Inherit: Inherit via back propagation  PCopyOutMin=[]  PCopyOutMax=[]  NCopyOutDataTypeStr=Inherit: Inherit via back propagation  NCopyOutMin=[]  NCopyOutMax=[]  IntegratorContinuousStateAttributes=''  IntegratorStateMustResolveToSignalObject=off  IntegratorRTWStateStorageClass=Auto  FilterContinuousStateAttributes=''  FilterStateMustResolveToSignalObject=off  FilterRTWStateStorageClass=Auto  ParallelPVariant=ExternalParameters  IdealPVariant=Disabled  IVariant=ExternalParameters  DVariant=ExternalParameters  IntegratorVariant=Discrete  SatVariant=Enabled  AWVariant=Passthrough  PCopyVariant=Disabled  TRVariant=Disabled  FdbkBlocksVariant=Forward  IdealPFdbkVariant=Disabled  SatFdbkVariant=Disabled  DerivativeFilterVariant=ForwardEulerFilter  NVariant=ExternalParameters  NCopyVariant=Disabled  FilterICVariant=InternalICsFilter  IntegratorICVariant=InternalICs  ExternalResetVariant=Disabled  TRSumVariant=Passthrough  SumFdbkVariant=Disabled  SumVariant=Sum_PID  TsampFilterVariant=InternalTs  TsampNgainVariant=Passthrough  TsampIntegralVariant=Disabled_SignalSpec  ExternalSaturationOutDataTypeStr=Inherit: Same as second input  DerivativeSourceVariant=ErrorSignal  PreIntVariant=InternalPreInt
  PID Controller4 : slpidlib/PID Controller  Controller=PID  Form=Parallel  TimeDomain=Discrete-time  UseExternalTs=off  SampleTime=-1  IntegratorMethod=Forward Euler  FilterMethod=Forward Euler  ControllerParametersSource=external  P=18.567926327114  I=2.74882046275699  UseKiTs=off  D=30.7980856287723  UseExternalDerivativeSource=off  N=17.2469682941307  UseFilter=on  TunerSelectOption=Transfer Function Based (PID Tuner App)  InitialConditionSource=internal  InitialConditionForIntegrator=0  InitialConditionForFilter=0  DifferentiatorICPrevScaledInput=0  ExternalReset=none  TrackingMode=off  Kt=1  LimitOutput=on  SatLimitsSource=internal  UpperSaturationLimit=max_yaw_torque  LowerSaturationLimit=-max_yaw_torque  LinearizeAsGain=on  AntiWindupMode=none  Kb=1  LimitIntegrator=off  UpperIntegratorSaturationLimit=inf  LowerIntegratorSaturationLimit=-inf  POutMin=[]  POutMax=[]  IOutMin=[]  IOutMax=[]  DOutMin=[]  DOutMax=[]  NOutMin=[]  NOutMax=[]  SumOutMin=[]  SumOutMax=[]  SaturationOutMin=[]  SaturationOutMax=[]  PParamMin=[]  PParamMax=[]  IParamMin=[]  IParamMax=[]  DParamMin=[]  DParamMax=[]  NParamMin=[]  NParamMax=[]  KbParamMin=[]  KbParamMax=[]  KtParamMin=[]  KtParamMax=[]  KbOutMin=[]  KbOutMax=[]  KtOutMin=[]  KtOutMax=[]  IntegratorOutMin=[]  IntegratorOutMax=[]  FilterOutMin=[]  FilterOutMax=[]  SumI1OutMin=[]  SumI1OutMax=[]  SumI2OutMin=[]  SumI2OutMax=[]  SumI3OutMin=[]  SumI3OutMax=[]  SumI4OutMin=[]  SumI4OutMax=[]  SumDOutMin=[]  SumDOutMax=[]  DifferentiatorOutMin=[]  DifferentiatorOutMax=[]  FilterDiffOutCoefMin=[]  FilterDiffOutCoefMax=[]  ReciprocalOutMin=[]  ReciprocalOutMax=[]  SumDenOutMin=[]  SumDenOutMax=[]  SumNumOutMin=[]  SumNumOutMax=[]  DivideOutMin=[]  DivideOutMax=[]  UdiffTsProdOutMin=[]  UdiffTsProdOutMax=[]  NTsProdOutMin=[]  NTsProdOutMax=[]  UintegralTsProdOutMin=[]  UintegralTsProdOutMax=[]  UngainTsProdOutMin=[]  UngainTsProdOutMax=[]  ClampingZeroOutDataTypeStr=Inherit: Inherit via back propagation  ClampingZeroOutMin=[]  ClampingZeroOutMax=[]  FilterDenConstantOutDataTypeStr=Inherit: Inherit via back propagation  FilterDenConstantOutMin=[]  FilterDenConstantOutMax=[]  PCopyOutDataTypeStr=Inherit: Inherit via back propagation  PCopyOutMin=[]  PCopyOutMax=[]  NCopyOutDataTypeStr=Inherit: Inherit via back propagation  NCopyOutMin=[]  NCopyOutMax=[]  IntegratorContinuousStateAttributes=''  IntegratorStateMustResolveToSignalObject=off  IntegratorRTWStateStorageClass=Auto  FilterContinuousStateAttributes=''  FilterStateMustResolveToSignalObject=off  FilterRTWStateStorageClass=Auto  ParallelPVariant=ExternalParameters  IdealPVariant=Disabled  IVariant=ExternalParameters  DVariant=ExternalParameters  IntegratorVariant=Discrete  SatVariant=Enabled  AWVariant=Passthrough  PCopyVariant=Disabled  TRVariant=Disabled  FdbkBlocksVariant=Forward  IdealPFdbkVariant=Disabled  SatFdbkVariant=Disabled  DerivativeFilterVariant=ForwardEulerFilter  NVariant=ExternalParameters  NCopyVariant=Disabled  FilterICVariant=InternalICsFilter  IntegratorICVariant=InternalICs  ExternalResetVariant=Disabled  TRSumVariant=Passthrough  SumFdbkVariant=Disabled  SumVariant=Sum_PID  TsampFilterVariant=InternalTs  TsampNgainVariant=Passthrough  TsampIntegralVariant=Disabled_SignalSpec  ExternalSaturationOutDataTypeStr=Inherit: Same as second input  DerivativeSourceVariant=ErrorSignal  PreIntVariant=InternalPreInt
  Position Selection : Selector  InputPortWidth=6  IndexOptions=Index vector (dialog)  Indices=[1:3]  OutputSizes=1
  To Workspace : ToWorkspace  VariableName=flags  SaveFormat=Timeseries  SampleTime=plot_dt
  Yaw Cross-Talk Corrector : MATLAB Function  TreatAsAtomicUnit=on
  Thruster Forces : Outport
  wires:
  Demux2/2 -> PID Controller/3
  Demux7/1 -> PID Controller4/2
  Gain Scheduler/1(xyz) -> Demux2/1
  PID Controller3/1 -> Mux/3
  state_error/1 -> Position Selection/1, Gain Scheduler/1(state_error), Attitude Selection/1
  PID Controller4/1 -> Mux/4
  Demux5/4 -> PID Controller2/5
  Mux/1 -> Thruster Forces/1
  PID Controller/1 -> Mux/1
  Demux5/2 -> PID Controller2/3
  Demux2/4 -> PID Controller/5
  Yaw Cross-Talk Corrector/1(corrected_error) -> PID Controller4/1
  Demux6/3 -> PID Controller3/4
  Demux2/1 -> PID Controller/2
  Demux6/4 -> PID Controller3/5
  Gain Scheduler/2(roll) -> Demux5/1
  Demux5/3 -> PID Controller2/4
  Demux6/1 -> PID Controller3/2
  Demux5/1 -> PID Controller2/2
  Demux6/2 -> PID Controller3/3
  Demux7/4 -> PID Controller4/5
  Demux7/2 -> PID Controller4/3
  Demux2/3 -> PID Controller/4
  Demux7/3 -> PID Controller4/4
  Gain Scheduler/3(pitch) -> Demux6/1
  Gain Scheduler/4(yaw) -> Demux7/1
  PID Controller2/1 -> Mux/2
  Position Selection/1 -> PID Controller/1
  Attitude Selection/1 -> Demux/1
  Demux/1 -> PID Controller2/1
  Demux/2 -> PID Controller3/1
  Demux/3 -> Yaw Cross-Talk Corrector/1(error)
  Data Store Read/1 -> To Workspace/1, Gain Scheduler/2("flags ")
  Gain Scheduler/5(flags) -> Data Store Write/1

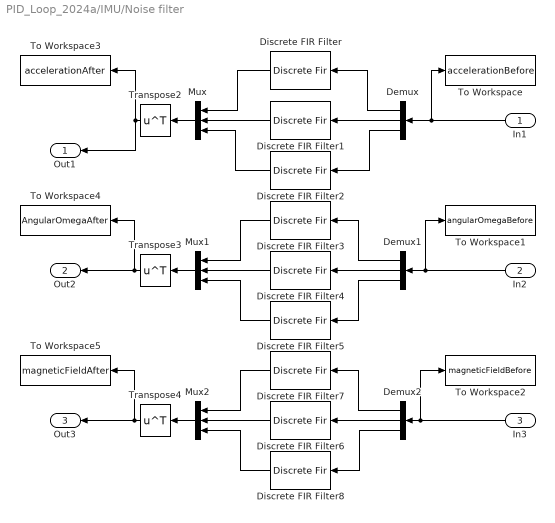
== system PID_Loop_2024a/IMU/Noise filter ==
  In1 : Inport
  In2 : Inport  Port=2
  In3 : Inport  Port=3
  Demux : Demux  Outputs=3
  Demux1 : Demux  Outputs=3
  Demux2 : Demux  Outputs=3
  Discrete FIR Filter{,1..5} (6 alike) : DiscreteFir  Coefficients=ones(1,15) / 15
  Discrete FIR Filter6 : DiscreteFir  Coefficients=ones(1,20) / 20
  Discrete FIR Filter7 : DiscreteFir  Coefficients=ones(1,20) / 20
  Discrete FIR Filter8 : DiscreteFir  Coefficients=ones(1,20) / 20
  Mux : Mux  Inputs=3
  Mux1 : Mux  Inputs=3
  Mux2 : Mux  Inputs=3
  To Workspace : ToWorkspace  VariableName=accelerationBefore  SaveFormat=Timeseries  SampleTime=-1
  To Workspace1 : ToWorkspace  VariableName=angularOmegaBefore  SaveFormat=Timeseries  SampleTime=-1
  To Workspace2 : ToWorkspace  VariableName=magneticFieldBefore  SaveFormat=Timeseries  SampleTime=-1
  To Workspace3 : ToWorkspace  VariableName=accelerationAfter  SaveFormat=Timeseries  SampleTime=-1
  To Workspace4 : ToWorkspace  VariableName=AngularOmegaAfter  SaveFormat=Timeseries  SampleTime=-1
  To Workspace5 : ToWorkspace  VariableName=magneticFieldAfter  SaveFormat=Timeseries  SampleTime=-1
  Transpose2 : Math  Operator=transpose
  Transpose3 : Math  Operator=transpose
  Transpose4 : Math  Operator=transpose
  Out1 : Outport
  Out2 : Outport  Port=2
  Out3 : Outport  Port=3
  wires:
  Mux1/1 -> Transpose3/1
  Discrete FIR Filter7/1 -> Mux2/1
  Mux/1 -> Transpose2/1
  Transpose2/1 -> To Workspace3/1, Out1/1
  Discrete FIR Filter6/1 -> Mux2/2
  Discrete FIR Filter5/1 -> Mux1/3
  In1/1 -> Demux/1, To Workspace/1
  In2/1 -> To Workspace1/1, Demux1/1
  Demux/1 -> Discrete FIR Filter/1
  Mux2/1 -> Transpose4/1
  Demux2/3 -> Discrete FIR Filter8/1
  Discrete FIR Filter1/1 -> Mux/2
  In3/1 -> To Workspace2/1, Demux2/1
  Discrete FIR Filter2/1 -> Mux/3
  Demux2/1 -> Discrete FIR Filter7/1
  Discrete FIR Filter8/1 -> Mux2/3
  Transpose3/1 -> Out2/1, To Workspace4/1
  Demux/3 -> Discrete FIR Filter2/1
  Discrete FIR Filter/1 -> Mux/1
  Demux/2 -> Discrete FIR Filter1/1
  Transpose4/1 -> Out3/1, To Workspace5/1
  Demux1/2 -> Discrete FIR Filter4/1
  Discrete FIR Filter4/1 -> Mux1/2
  Demux2/2 -> Discrete FIR Filter6/1
  Discrete FIR Filter3/1 -> Mux1/1
  Demux1/3 -> Discrete FIR Filter5/1
  Demux1/1 -> Discrete FIR Filter3/1

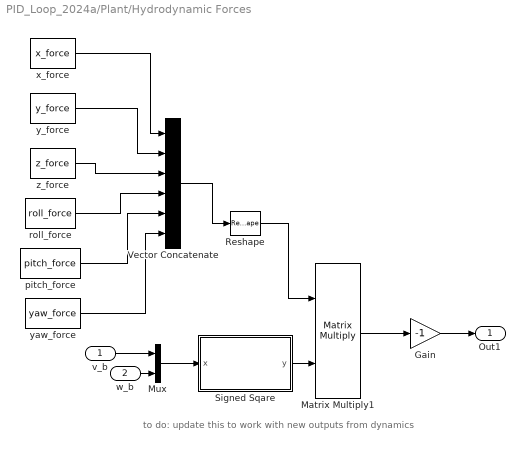
== system PID_Loop_2024a/Plant/Hydrodynamic Forces ==
  note: to do: update this to work with new outputs from dynamics
  v_b : Inport
  w_b : Inport  Port=2
  Gain : Gain  Gain=-1
  Matrix Multiply1 : Product  Multiplication=Matrix(*)
  Mux : Mux  Inputs=2
  Reshape : Reshape  OutputDimensionality=Customize  OutputDimensions=[6,6]
  Signed Sqare : MATLAB Function  TreatAsAtomicUnit=on
  Vector Concatenate : Concatenate  NumInputs=6
  pitch_force : Constant  Value=pitch_force  VectorParams1D=off
  roll_force : Constant  Value=roll_force  VectorParams1D=off
  x_force : Constant  Value=x_force  VectorParams1D=off
  y_force : Constant  Value=y_force  VectorParams1D=off
  yaw_force : Constant  Value=yaw_force  VectorParams1D=off
  z_force : Constant  Value=z_force  VectorParams1D=off
  Out1 : Outport
  wires:
  Matrix Multiply1/1 -> Gain/1
  Signed Sqare/1(y) -> Matrix Multiply1/2
  Gain/1 -> Out1/1
  Mux/1 -> Signed Sqare/1(x)
  v_b/1 -> Mux/1
  w_b/1 -> Mux/2
  Reshape/1 -> Matrix Multiply1/1
  x_force/1 -> Vector Concatenate/1
  y_force/1 -> Vector Concatenate/2
  z_force/1 -> Vector Concatenate/3
  roll_force/1 -> Vector Concatenate/4
  pitch_force/1 -> Vector Concatenate/5
  yaw_force/1 -> Vector Concatenate/6
  Vector Concatenate/1 -> Reshape/1

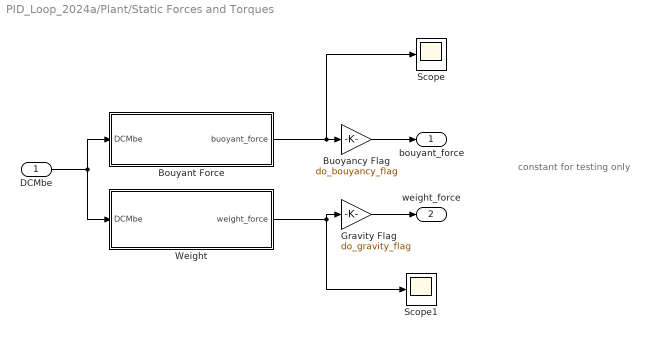
== system PID_Loop_2024a/Plant/Static Forces and Torques ==
  note: constant for testing only
  DCMbe : Inport
  Bouyant Force : MATLAB Function  TreatAsAtomicUnit=on
  Buoyancy Flag : Gain  Gain=do_bouyancy_flag
  Gravity Flag : Gain  Gain=do_gravity_flag
  Scope : Scope
  Scope1 : Scope
  Weight : MATLAB Function  TreatAsAtomicUnit=on
  bouyant_force : Outport
  weight_force : Outport  Port=2
  wires:
  DCMbe/1 -> Weight/1(DCMbe), Bouyant Force/1(DCMbe)
  Buoyancy Flag/1 -> bouyant_force/1
  Gravity Flag/1 -> weight_force/1
  Weight/1(weight_force) -> Gravity Flag/1, Scope1/1
  Bouyant Force/1(buoyant_force) -> Scope/1, Buoyancy Flag/1

== system PID_Loop_2024a/Plant/Thruster Forces ==
  thruster_pwms : Inport
  PWM to Motor Forces : MATLAB Function  TreatAsAtomicUnit=on
  Product : Product  Multiplication=Matrix(*)
  Scope : Scope
  To Workspace : ToWorkspace  VariableName=thruster_delivered  SaveFormat=Timeseries  SampleTime=plot_dt
  To Workspace4 : ToWorkspace  VariableName=force_torque_delivered  SaveFormat=Timeseries  SampleTime=plot_dt
  Wrench Matrix : Constant  Value=wrench  VectorParams1D=off
  thruster forces and moments : Outport
  wires:
  Product/1 -> To Workspace4/1, thruster forces and moments/1
  thruster_pwms/1 -> PWM to Motor Forces/1(thruster_pwms)
  Wrench Matrix/1 -> Product/1
  PWM to Motor Forces/1(forces_N) -> Product/2, Scope/1, To Workspace/1

== system PID_Loop_2024a/SPU/Temporary Brute Force Integration ==
  w_b_imu : Inport
  A_be_imu : Inport  Port=2
  Integrator : Integrator  InitialCondition=v0_e_est
  Integrator1 : Integrator  InitialCondition=x0_e_est
  Integrator2 : Integrator  InitialCondition=E0_est
  Inverted Attitude Kinematics : MATLAB Function  TreatAsAtomicUnit=on
  x_e_est : Outport
  E_est : Outport  Port=2
  wires:
  A_be_imu/1 -> Integrator/1
  Integrator/1 -> Integrator1/1
  w_b_imu/1 -> Inverted Attitude Kinematics/1(w_est)
  Inverted Attitude Kinematics/1(dE_est) -> Integrator2/1
  Integrator2/1 -> E_est/1, Inverted Attitude Kinematics/2(E_est)
  Integrator1/1 -> x_e_est/1

== matlab function PID_Loop_2024a/MATLAB Function1 ==
  data: t input; y output
function y = fcn(t)

if t < 30
    y = t;
elseif t < 60
    y = 30;
else
    y = 90 - t;

end

== matlab function PID_Loop_2024a/Attitude EKF/Measure Eulers ==
  data: phi_meas output; Abe_b input; theta_meas output; m_b input; psi_meas output
function [phi_meas, theta_meas, psi_meas] = fcn(Abe_b,m_b)

%This function calculates the attitude of the vehicle using the
%acceleration vector direction and the magnetic field vector direction
%based on the assumption that the only acceleration is gravity in the
%inertial up (+z) direction and the magnetic field points in the inertial north
%(+x).

%unpack input
ax = Abe_b(1);
ay = Abe_b(2);
az = Abe_b(3);
mx = m_b(1);
my = m_b(2);


theta_meas = atan2((-ax), sqrt(ay*ay + az*az));
phi_meas = atan2(ay,az);
psi_meas = atan2(-my, mx);

== matlab function PID_Loop_2024a/Controller/6 DOF Gain Scheduled PID/Gain Scheduler ==
  data: state_error input; xyz output; roll output; pitch output; yaw output; flags input; flags output
%The goal is to take state errors, determine the most desired state which
%we want to control. And then determine the gains to optimize that state
%control.

% If(roll error > Some saturation value)

%Yaw should have a much smaller error for this code architecture, we want
%to be pretty accurate

function[xyz, roll, pitch, yaw,flags] = gainScheduler(state_error,flags)

%unpack flags
roll_flag = flags(1);
pitch_flag = flags(2);
yaw_flag = flags(3);

roll_err = state_error(4); %Phi
pitch_err = state_error(5); %Theta
yaw_err = state_error(6); %Psi

%% Upper and Lower error bounds for control

%gain scheduling parameters
roll_upper = 5*pi/180;
roll_lower = 1*pi/180;
pitch_upper = 5*pi/180;
pitch_lower = 1*pi/180;
yaw_upper = 5*pi/180;
yaw_lower = 1*pi/180;




%% Roll, Pitch, and Yaw Flaggers
if(abs(yaw_err) >= yaw_upper)
    yaw_flag = 1;
elseif(abs(yaw_err) < yaw_lower)
    yaw_flag = 0;
else
    yaw_flag = yaw_flag;
end

if(abs(pitch_err) >= pitch_upper)
    pitch_flag = 1;
    yaw_flag = 0;
elseif(abs(pitch_err) < pitch_lower)
    pitch_flag = 0;
else
    pitch_flag = pitch_flag;
    yaw_flag = 0;
end

if(abs(roll_err) >= roll_upper)
    roll_flag = 1;
    yaw_flag = 0;
elseif(abs(roll_err) < roll_lower)
    roll_flag = 0;
else
    roll_flag = roll_flag;
    yaw_flag = 0;
end


%% Scheduler


%Roll, Pitch, and Yaw Scheduling
if((roll_flag == 1) || (pitch_flag == 1))
    %don't want position and yaw control here
    roll = [4.773, 2.325 , 2.504, 54.540];
    pitch = [6.912, 3.236 , 3.625, 54.540];
    yaw = 0*[6.782, 2.479, 2.957, 1142.828];
    xyz = [0 0 0 1];
elseif(yaw_flag == 1)
    %do yaw control if pitch and roll are ok
    yaw = [6.782, 2.479, 2.957, 1142.828];
    roll = [4.773, 2.325 , 2.504, 54.540];
    pitch = [6.912, 3.236 , 3.625, 54.540];
    xyz = [0 0 0 1];
else
    %do position control, ok to leave on roll pitch and yaw because error
    %should be small
    xyz = [18.568, 2.749, 30.798, 17.247];
    roll = [4.773, 2.325 , 2.504, 54.540];
    pitch = [6.912, 3.236 , 3.625, 54.540];
    yaw = [6.782, 2.479, 2.957, 1142.828];
    
end

%pack up flags
flags = [roll_flag,pitch_flag,yaw_flag]';
end

== matlab function PID_Loop_2024a/MATLAB Function8 ==
  data: t input; y output
function y = fcn(t)

speed = 30 / 30; 
if t < 30
    y = 0;
elseif t < 60
    y = 30 * speed - t * speed;
else
    y = 30 * speed - 60 * speed;
end

== matlab function PID_Loop_2024a/Controller/6 DOF Gain Scheduled PID/Yaw Cross-Talk Corrector ==
  data: error input; corrected_error output
function corrected_error = fcn(error)
    if(error > 180)
        corrected_error = error - 360;
    elseif(error < -180)
        corrected_error = error + 360;
    else
        corrected_error = error;
    end
end

== matlab function PID_Loop_2024a/SPU/MATLAB Function ==
  data: input input; output output
function output = fcn(input)
%#codegen
e = exp(1);
%Ok the cutoff frequency would be 2000 Hz
alpha = e^(-2 * pi * (2000/8000));
N = length(input);
myFourier = fft(input);
omega = 2 * pi * (0:N-1)' / N;
    transformFunction = (1- alpha) ./ (1 - alpha * e^(-1i * omega));
    transformedSignal = myFourier .* transformFunction;
    output = ifft(transformedSignal);

== matlab function PID_Loop_2024a/SPU/MATLAB Function1 ==
  data: input input; output output
function output = fcn(input)
%#codegen
e = exp(1);
%Ok the cutoff frequency would be 2000 Hz
alpha = e^(-2 * pi * (2000/8000));
N = length(input);
myFourier = fft(input);
omega = 2 * pi * (0:N-1)' / N;
    transformFunction = (1- alpha) ./ (1 - alpha * e^(-1i * omega));
    transformedSignal = myFourier .* transformFunction;
    output = ifft(transformedSignal);

== matlab function PID_Loop_2024a/Plant/Hydrodynamic Forces/Signed Sqare ==
  data: x input; y output
function y = signed_square(x)
y = x .* abs(x);
end
